simulink library "RxTxFixedPointLibrary_noscopes_org"  (Simulink 10.0)
settings: Solver=VariableStepAuto  StartTime=0.0  StopTime=10.0  RelTol=1e-3
undefined symbols (not defined in the file): AGCBarkerSymbols, coeff, crcDecodeLag, CRCGeneratorLag, EQTrainingSymbols, j, K1, K2, numHeaderBits, numTrainingSamples, pLen, RadioSampleRate, samplesPerSymbol, VibertiTracebackLength, xPreambleSeq
libraries: simulink x33, dsphdlfiltering x20, hdlsllib x13, commseqgen3 x4, dspsigops x4, commdigbbndpm3 x3, commcrc2 x2, commcnvcod2 x2, $bdroot x1, dspstat3 x1, commfilt2 x1
(part 1 of 4)
settings Model: Creator=tcollins  LastModifiedBy=annonymous
settings Model: SuppressorTable=|
  | <?xml version="1.0" encoding="UTF-8" standalone="yes" ?>
  | <!DOCTYPE boost_serialization>
  | <boost_serialization signature="serialization::archive" version="15">
  | <DiagnosticSuppressor class_id="0" tracking_level="0" version="6">
  | 	<Table class_id="1" tracking_level="0" version="0">
  | 		<count>28</count>
  | 		<bucket_count>47</bucket_count>
  | 		<item_version>0</item_version>
  | 		<item class_id="2" tracking_level="0" version="0">
  | 			<first class_id="3" tracking_level="0" version="6">
  | 				<Source class_id="4" tracking_level="0" version="0">
  | 					<count>1</count>
  | 					<item_version>0</item_version>
  | 					<item>RxTxFixedPointLibrary_noscopes_org/Receiver HDL/Frame Recover/Frequency Recovery/Phase Shift FP/Cosine HDL Optimized</item>
  | 				</Source>
  | 			</first>
  | 			<second class_id="5" tracking_level="0" version="6">
  | 				<SuppressedData class_id="6" tracking_level="0" version="0">
  | 					<count>1</count>
  | 					<bucket_count>2</bucket_count>
  | 					<item_version>0</item_version>
  | 					<item class_id="7" tracking_level="0" version="0">
  | 						<first class_id="8" tracking_level="0" version="6">
  | 							<ID>SimulinkFixedPoint:util:fxpParameterPrecisionLoss</ID>
  | 							<Cause>
  | 								<Source>
  | 									<count>0</count>
  | 									<item_version>0</item_version>
  | 								</Source>
  | 							</Cause>
  | 						</first>
  | 						<second class_id="9" tracking_level="0" version="6">
  | 							<Comment></Comment>
  | 							<User></User>
  | 							<LastModified class_id="10" tracking_level="0" version="0">
  | 								<ptime_date class_id="11" tracking_level="0" version="0">
  | 									<date>20160608</date>
  | 								</ptime_date>
  | 								<ptime_time_duration class_id="12" tracking_level="0" version="0">
  | 									<is_special>0</is_special>
  | 									<time_duration_hours>12</time_duration_hours>
  | 									<time_duration_minutes>6</time_duration_minutes>
  | 									<time_duration_seconds>23</time_duration_seconds>
  | 									<time_duration_fractional_seconds>0</time_duration_fractional_seconds>
  | 								</ptime_time_duration>
  | 							</LastModified>
  | 							<SuppressionType>1</SuppressionType>
  | 						</second>
  | 					</item>
  | 				</SuppressedData>
  | 			</second>
  | 		</item>
  | 		<item>
  | 			<first>
  | 				<Source>
  | 					<count>1</count>
  | 					<item_version>0</item_version>
  | 					<item>RxTxFixedPointLibrary_noscopes_org/Receiver HDL/Viterbi Decode/Buffer Frame/FIFO/HDL FIFO4/Upsample2/Counter</item>
  | 				</Source>
  | 			</first>
  | 			<second>
  | 				<SuppressedData>
  | 					<count>2</count>
  | 					<bucket_count>2</bucket_count>
  | 					<item_version>0</item_version>
  | 					<item>
  | 						<first>
  | 							<ID>SimulinkFixedPoint:util:Overflowoccurred</ID>
  | 							<Cause>
  | 								<Source>
  | 									<count>0</count>
  | 									<item_version>0</item_version>
  | 								</Source>
  | 							</Cause>
  | 						</first>
  | 						<second>
  | 							<Comment></Comment>
  | 							<User></User>
  | 							<LastModified>
  | 								<ptime_date>
  | 									<date>20160608</date>
  | 								</ptime_date>
  | 								<ptime_time_duration>
  | 									<is_special>0</is_special>
  | 									<time_duration_hours>15</time_duration_hours>
  | 									<time_duration_minutes>23</time_duration_minutes>
  | 									<time_duration_seconds>17</time_duration_seconds>
  | 									<time_duration_fractional_seconds>0</time_duration_fractional_seconds>
  | 								</ptime_time_duration>
  | 							</LastModified>
  | 							<SuppressionType>1</SuppressionType>
  | 						</second>
  | 					</item>
  | 					<item>
  | 						<first>
  | 							<ID>Simulink:DataType:WarningOverFlowDetected</ID>
  | 							<Cause>
  | 								<Source>
  | 									<count>0</count>
  | 									<item_version>0</item_version>
  | 								</Source>
  | 							</Cause>
  | 						</first>
  | 						<second>
  | 							<Comment></Comment>
  | 							<User></User>
  | 							<LastModified>
  | 								<ptime_date>
  | 									<date>20160608</date>
  | 								</ptime_date>
  | 								<ptime_time_duration>
  | 									<is_special>0</is_special>
  | 									<time_duration_hours>15</time_duration_hours>
  | 									<time_duration_minutes>23</time_duration_minutes>
  | 									<time_duration_seconds>17</time_duration_seconds>
  | 									<time_duration_fractional_seconds>0</time_duration_fractional_seconds>
  | 								</ptime_time_duration>
  | 							</LastModified>
  | 							<SuppressionType>1</SuppressionType>
  | 						</second>
  | 					</item>
  | 				</SuppressedData>
  | 			</second>
  | 		</item>
  | 		<item>
  | 			<first>
  | 				<Source>
  | 					<count>1</count>
  | 					<item_version>0</item_version>
  | 					<item>RxTxFixedPointLibrary_noscopes_org/Transmitter HDL/Packet Generation/Frame Indexer</item>
  | 				</Source>
  | 			</first>
  | 			<second>
  | 				<SuppressedData>
  | 					<count>2</count>
  | 					<bucket_count>2</bucket_count>
  | 					<item_version>0</item_version>
  | 					<item>
  | 						<first>
  | 							<ID>Simulink:DataType:WarningOverFlowDetected</ID>
  | 							<Cause>
  | 								<Source>
  | 									<count>0</count>
  | 									<item_version>0</item_version>
  | 								</Source>
  | 							</Cause>
  | 						</first>
  | 						<second>
  | 							<Comment></Comment>
  | 							<User></User>
  | 							<LastModified>
  | 								<ptime_date>
  | 									<date>20160715</date>
  | 								</ptime_date>
  | 								<ptime_time_duration>
  | 									<is_special>0</is_special>
  | 									<time_duration_hours>14</time_duration_hours>
  | 									<time_duration_minutes>21</time_duration_minutes>
  | 									<time_duration_seconds>36</time_duration_seconds>
  | 									<time_duration_fractional_seconds>0</time_duration_fractional_seconds>
  | 								</ptime_time_duration>
  | 							</LastModified>
  | 							<SuppressionType>1</SuppressionType>
  | 						</second>
  | 					</item>
  | 					<item>
  | 						<first>
  | 							<ID>SimulinkFixedPoint:util:Overflowoccurred</ID>
  | 							<Cause>
  | 								<Source>
  | 									<count>0</count>
  | 									<item_version>0</item_version>
  | 								</Source>
  | 							</Cause>
  | 						</first>
  | 						<second>
  | 							<Comment></Comment>
  | 							<User></User>
  | 							<LastModified>
  | 								<ptime_date>
  | 									<date>20160715</date>
  | 								</ptime_date>
  | 								<ptime_time_duration>
  | 									<is_special>0</is_special>
  | 									<time_duration_hours>14</time_duration_hours>
  | 									<time_duration_minutes>21</time_duration_minutes>
  | 									<time_duration_seconds>36</time_duration_seconds>
  | 									<time_duration_fractional_seconds>0</time_duration_fractional_seconds>
  | 								</ptime_time_duration>
  | 							</LastModified>
  | 							<SuppressionType>1</SuppressionType>
  | 						</second>
  | 					</item>
  | 				</SuppressedData>
  | 			</second>
  | 		</item>
  | 		<item>
  | 			<first>
  | 				<Source>
  | 					<count>1</count>
  | 					<item_version>0</item_version>
  | 					<item>RxTxFixedPointLibrary_noscopes_org/Receiver HDL/Frame Recover/Frequency Recovery/Phase Shift FP/Cosine HDL Optimized/exp hdl/cos_hdl</item>
  | 				</Source>
  | 			</first>
  | 			<second>
  | 				<SuppressedData>
  | 					<count>1</count>
  | 					<bucket_count>2</bucket_count>
  | 					<item_version>0</item_version>
  | 					<item>
  | 						<first>
  | 							<ID>SimulinkFixedPoint:util:fxpParameterPrecisionLoss</ID>
  | 							<Cause>
  | 								<Source>
  | 									<count>0</count>
  | 									<item_version>0</item_version>
  | 								</Source>
  | 							</Cause>
  | 						</first>
  | 						<second>
  | 							<Comment></Comment>
  | 							<User></User>
  | 							<LastModified>
  | 								<ptime_date>
  | 									<date>20160607</date>
  | 								</ptime_date>
  | 								<ptime_time_duration>
  | 									<is_special>0</is_special>
  | 									<time_duration_hours>13</time_duration_hours>
  | 									<time_duration_minutes>40</time_duration_minutes>
  | 									<time_duration_seconds>47</time_duration_seconds>
  | 									<time_duration_fractional_seconds>0</time_duration_fractional_seconds>
  | 								</ptime_time_duration>
  | 							</LastModified>
  | 							<SuppressionType>1</SuppressionType>
  | 						</second>
  | 					</item>
  | 				</SuppressedData>
  | 			</second>
  | 		</item>
  | 		<item>
  | 			<first>
  | 				<Source>
  | 					<count>1</count>
  | 					<item_version>0</item_version>
  | 					<item>RxTxFixedPointLibrary_noscopes_org/Receiver HDL/Frame Recover/Frequency Recovery/Phase Shift FP/Cosine HDL Optimized/exp hdl/sin_hdl/CastU16En3</item>
  | 				</Source>
  | 			</first>
  | 			<second>
  | 				<SuppressedData>
  | 					<count>1</count>
  | 					<bucket_count>2</bucket_count>
  | 					<item_version>0</item_version>
  | 					<item>
  | 						<first>
  | 							<ID>SimulinkFixedPoint:util:Saturationoccurred</ID>
  | 							<Cause>
  | 								<Source>
  | 									<count>0</count>
  | 									<item_version>0</item_version>
  | 								</Source>
  | 							</Cause>
  | 						</first>
  | 						<second>
  | 							<Comment></Comment>
  | 							<User>sdutta</User>
  | 							<LastModified>
  | 								<ptime_date>
  | 									<date>20170912</date>
  | 								</ptime_date>
  | 								<ptime_time_duration>
  | 									<is_special>0</is_special>
  | 									<time_duration_hours>16</time_duration_hours>
  | 									<time_duration_minutes>2</time_duration_minutes>
  | 									<time_duration_seconds>5</time_duration_seconds>
  | 									<time_duration_fractional_seconds>0</time_duration_fractional_seconds>
  | 								</ptime_time_duration>
  | 							</LastModified>
  | 							<SuppressionType>1</SuppressionType>
  | 						</second>
  | 					</item>
  | 				</SuppressedData>
  | 			</second>
  | 		</item>
  | 		<item>
  | 			<first>
  | 				<Source>
  | 					<count>1</count>
  | 					<item_version>0</item_version>
  | 					<item>RxTxFixedPointLibrary_noscopes_org/Transmitter HDL/Packet Generation/Random Data/Unpack/Extract Bits</item>
  | 				</Source>
  | 			</first>
  | 			<second>
  | 				<SuppressedData>
  | 					<count>2</count>
  | 					<bucket_count>2</bucket_count>
  | 					<item_version>0</item_version>
  | 					<item>
  | 						<first>
  | 							<ID>SimulinkFixedPoint:util:Overflowoccurred</ID>
  | 							<Cause>
  | 								<Source>
  | 									<count>0</count>
  | 									<item_version>0</item_version>
  | 								</Source>
  | 							</Cause>
  | 						</first>
  | 						<second>
  | 							<Comment></Comment>
  | 							<User></User>
  | 							<LastModified>
  | 								<ptime_date>
  | 									<date>20160608</date>
  | 								</ptime_date>
  | 								<ptime_time_duration>
  | 									<is_special>0</is_special>
  | 									<time_duration_hours>15</time_duration_hours>
  | 									<time_duration_minutes>43</time_duration_minutes>
  | 									<time_duration_seconds>6</time_duration_seconds>
  | 									<time_duration_fractional_seconds>0</time_duration_fractional_seconds>
  | 								</ptime_time_duration>
  | 							</LastModified>
  | 							<SuppressionType>1</SuppressionType>
  | 						</second>
  | 					</item>
  | 					<item>
  | 						<first>
  | 							<ID>Simulink:DataType:WarningOverFlowDetected</ID>
  | 							<Cause>
  | 								<Source>
  | 									<count>0</count>
  | 									<item_version>0</item_version>
  | 								</Source>
  | 							</Cause>
  | 						</first>
  | 						<second>
  | 							<Comment></Comment>
  | 							<User></User>
  | 							<LastModified>
  | 								<ptime_date>
  | 									<date>20160608</date>
  | 								</ptime_date>
  | 								<ptime_time_duration>
  | 									<is_special>0</is_special>
  | 									<time_duration_hours>15</time_duration_hours>
  | 									<time_duration_minutes>43</time_duration_minutes>
  | 									<time_duration_seconds>6</time_duration_seconds>
  | 									<time_duration_fractional_seconds>0</time_duration_fractional_seconds>
  | 								</ptime_time_duration>
  | 							</LastModified>
  | 							<SuppressionType>1</SuppressionType>
  | 						</second>
  | 					</item>
  | 				</SuppressedData>
  | 			</second>
  | 		</item>
  | 		<item>
  | 			<first>
  | 				<Source>
  | 					<count>1</count>
  | 					<item_version>0</item_version>
  | 					<item>RxTxFixedPointLibrary_noscopes_org/Receiver HDL/Frame Recover/Equalization and Demodulation/DFE/DFE/Map Symbol/HDL Counter</item>
  | 				</Source>
  | 			</first>
  | 			<second>
  | 				<SuppressedData>
  | 					<count>2</count>
  | 					<bucket_count>2</bucket_count>
  | 					<item_version>0</item_version>
  | 					<item>
  | 						<first>
  | 							<ID>Simulink:DataType:WarningOverFlowDetected</ID>
  | 							<Cause>
  | 								<Source>
  | 									<count>0</count>
  | 									<item_version>0</item_version>
  | 								</Source>
  | 							</Cause>
  | 						</first>
  | 						<second>
  | 							<Comment></Comment>
  | 							<User></User>
  | 							<LastModified>
  | 								<ptime_date>
  | 									<date>20160715</date>
  | 								</ptime_date>
  | 								<ptime_time_duration>
  | 									<is_special>0</is_special>
  | 									<time_duration_hours>14</time_duration_hours>
  | 									<time_duration_minutes>21</time_duration_minutes>
  | 									<time_duration_seconds>36</time_duration_seconds>
  | 									<time_duration_fractional_seconds>0</time_duration_fractional_seconds>
  | 								</ptime_time_duration>
  | 							</LastModified>
  | 							<SuppressionType>1</SuppressionType>
  | 						</second>
  | 					</item>
  | 					<item>
  | 						<first>
  | 							<ID>SimulinkFixedPoint:util:Overflowoccurred</ID>
  | 							<Cause>
  | 								<Source>
  | 									<count>0</count>
  | 									<item_version>0</item_version>
  | 								</Source>
  | 							</Cause>
  | 						</first>
  | 						<second>
  | 							<Comment></Comment>
  | 							<User></User>
  | 							<LastModified>
  | 								<ptime_date>
  | 									<date>20160715</date>
  | 								</ptime_date>
  | 								<ptime_time_duration>
  | 									<is_special>0</is_special>
  | 									<time_duration_hours>14</time_duration_hours>
  | 									<time_duration_minutes>21</time_duration_minutes>
  | 									<time_duration_seconds>36</time_duration_seconds>
  | 									<time_duration_fractional_seconds>0</time_duration_fractional_seconds>
  | 								</ptime_time_duration>
  | 							</LastModified>
  | 							<SuppressionType>1</SuppressionType>
  | 						</second>
  | 					</item>
  | 				</SuppressedData>
  | 			</second>
  | 		</item>
  | 		<item>
  | 			<first>
  | 				<Source>
  | 					<count>1</count>
  | 					<item_version>0</item_version>
  | 					<item>RxTxFixedPointLibrary_noscopes_org/Receiver HDL/Viterbi Decode/Buffer Frame/FIFO/HDL FIFO4/Upsample1/Counter</item>
  | 				</Source>
  | 			</first>
  | 			<second>
  | 				<SuppressedData>
  | 					<count>2</count>
  | 					<bucket_count>2</bucket_count>
  | 					<item_version>0</item_version>
  | 					<item>
  | 						<first>
  | 							<ID>SimulinkFixedPoint:util:Overflowoccurred</ID>
  | 							<Cause>
  | 								<Source>
  | 									<count>0</count>
  | 									<item_version>0</item_version>
  | 								</Source>
  | 							</Cause>
  | 						</first>
  | 						<second>
  | 							<Comment></Comment>
  | 							<User></User>
  | 							<LastModified>
  | 								<ptime_date>
  | 									<date>20160608</date>
  | 								</ptime_date>
  | 								<ptime_time_duration>
  | 									<is_special>0</is_special>
  | 									<time_duration_hours>15</time_duration_hours>
  | 									<time_duration_minutes>23</time_duration_minutes>
  | 									<time_duration_seconds>17</time_duration_seconds>
  | 									<time_duration_fractional_seconds>0</time_duration_fractional_seconds>
  | 								</ptime_time_duration>
  | 							</LastModified>
  | 							<SuppressionType>1</SuppressionType>
  | 						</second>
  | 					</item>
  | 					<item>
  | 						<first>
  | 							<ID>Simulink:DataType:WarningOverFlowDetected</ID>
  | 							<Cause>
  | 								<Source>
  | 									<count>0</count>
  | 									<item_version>0</item_version>
  | 								</Source>
  | 							</Cause>
  | 						</first>
  | 						<second>
  | 							<Comment></Comment>
  | 							<User></User>
  | 							<LastModified>
  | 								<ptime_date>
  | 									<date>20160608</date>
  | 								</ptime_date>
  | 								<ptime_time_duration>
  | 									<is_special>0</is_special>
  | 									<time_duration_hours>15</time_duration_hours>
  | 									<time_duration_minutes>23</time_duration_minutes>
  | 									<time_duration_seconds>17</time_duration_seconds>
  | 									<time_duration_fractional_seconds>0</time_duration_fractional_seconds>
  | 								</ptime_time_duration>
  | 							</LastModified>
  | 							<SuppressionType>1</SuppressionType>
  | 						</second>
  | 					</item>
  | 				</SuppressedData>
  | 			</second>
  | 		</item>
  | 		<item>
  | 			<first>
  | 				<Source>
  | 					<count>1</count>
  | 					<item_version>0</item_version>
  | 					<item>RxTxFixedPointLibrary_noscopes_org/Transmitter HDL/Packet Generation/Preamble/HDL Counter</item>
  | 				</Source>
  | 			</first>
  | 			<second>
  | 				<SuppressedData>
  | 					<count>2</count>
  | 					<bucket_count>2</bucket_count>
  | 					<item_version>0</item_version>
  | 					<item>
  | 						<first>
  | 							<ID>Simulink:DataType:WarningOverFlowDetected</ID>
  | 							<Cause>
  | 								<Source>
  | 									<count>0</count>
  | 									<item_version>0</item_version>
  | 								</Source>
  | 							</Cause>
  | 						</first>
  | 						<second>
  | 							<Comment></Comment>
  | 							<User></User>
  | 							<LastModified>
  | 								<ptime_date>
  | 									<date>20160715</date>
  | 								</ptime_date>
  | 								<ptime_time_duration>
  | 									<is_special>0</is_special>
  | 									<time_duration_hours>14</time_duration_hours>
  | 									<time_duration_minutes>21</time_duration_minutes>
  | 									<time_duration_seconds>36</time_duration_seconds>
  | 									<time_duration_fractional_seconds>0</time_duration_fractional_seconds>
  | 								</ptime_time_duration>
  | 							</LastModified>
  | 							<SuppressionType>1</SuppressionType>
  | 						</second>
  | 					</item>
  | 					<item>
  | 						<first>
  | 							<ID>SimulinkFixedPoint:util:Overflowoccurred</ID>
  | 							<Cause>
  | 								<Source>
  | 									<count>0</count>
  | 									<item_version>0</item_version>
  | 								</Source>
  | 							</Cause>
  | 						</first>
  | 						<second>
  | 							<Comment></Comment>
  | 							<User></User>
  | 							<LastModified>
  | 								<ptime_date>
  | 									<date>20160715</date>
  | 								</ptime_date>
  | 								<ptime_time_duration>
  | 									<is_special>0</is_special>
  | 									<time_duration_hours>14</time_duration_hours>
  | 									<time_duration_minutes>21</time_duration_minutes>
  | 									<time_duration_seconds>36</time_duration_seconds>
  | 									<time_duration_fractional_seconds>0</time_duration_fractional_seconds>
  | 								</ptime_time_duration>
  | 							</LastModified>
  | 							<SuppressionType>1</SuppressionType>
  | 						</second>
  | 					</item>
  | 				</SuppressedData>
  | 			</second>
  | 		</item>
  | 		<item>
  | 			<first>
  | 				<Source>
  | 					<count>1</count>
  | 					<item_version>0</item_version>
  | 					<item>RxTxFixedPointLibrary_noscopes_org/Transmitter HDL/Packet Generation/Random Data/Unpack/Extract Bits1</item>
  | 				</Source>
  | 			</first>
  | 			<second>
  | 				<SuppressedData>
  | 					<count>2</count>
  | 					<bucket_count>2</bucket_count>
  | 					<item_version>0</item_version>
  | 					<item>
  | 						<first>
  | 							<ID>SimulinkFixedPoint:util:Overflowoccurred</ID>
  | 							<Cause>
  | 								<Source>
  | 									<count>0</count>
  | 									<item_version>0</item_version>
  | 								</Source>
  | 							</Cause>
  | 						</first>
  | 						<second>
  | 							<Comment></Comment>
  | 							<User></User>
  | 							<LastModified>
  | 								<ptime_date>
  | 									<date>20160608</date>
  | 								</ptime_date>
  | 								<ptime_time_duration>
  | 									<is_special>0</is_special>
  | 									<time_duration_hours>15</time_duration_hours>
  | 									<time_duration_minutes>43</time_duration_minutes>
  | 									<time_duration_seconds>6</time_duration_seconds>
  | 									<time_duration_fractional_seconds>0</time_duration_fractional_seconds>
  | 								</ptime_time_duration>
  | 							</LastModified>
  | 							<SuppressionType>1</SuppressionType>
  | 						</second>
  | 					</item>
  | 					<item>
  | 						<first>
  | 							<ID>Simulink:DataType:WarningOverFlowDetected</ID>
  | 							<Cause>
  | 								<Source>
  | 									<count>0</count>
  | 									<item_version>0</item_version>
  | 								</Source>
  | 							</Cause>
  | 						</first>
  | 						<second>
  | 							<Comment></Comment>
  | 							<User></User>
  | 							<LastModified>
  | 								<ptime_date>
  | 									<date>20160608</date>
  | 								</ptime_date>
  | 								<ptime_time_duration>
  | 									<is_special>0</is_special>
  | 									<time_duration_hours>15</time_duration_hours>
  | 									<time_duration_minutes>43</time_duration_minutes>
  | 									<time_duration_seconds>6</time_duration_seconds>
  | 									<time_duration_fractional_seconds>0</time_duration_fractional_seconds>
  | 								</ptime_time_duration>
  | 							</LastModified>
  | 							<SuppressionType>1</SuppressionType>
  | 						</second>
  | 					</item>
  | 				</SuppressedData>
  | 			</second>
  | 		</item>
  | 		<item>
  | 			<first>
  | 				<Source>
  | 					<count>1</count>
  | 					<item_version>0</item_version>
  | 					<item>RxTxFixedPointLibrary_noscopes_org/Receiver HDL/Frame Recover/Frequency Recovery/Phase Shift FP/Cosine HDL Optimized/exp hdl/sin_hdl/insig</item>
  | 				</Source>
  | 			</first>
  | 			<second>
  | 				<SuppressedData>
  | 					<count>1</count>
  | 					<bucket_count>2</bucket_count>
  | 					<item_version>0</item_version>
  | 					<item>
  | 						<first>
  | 							<ID>SimulinkFixedPoint:util:Overflowoccurred</ID>
  | 							<Cause>
  | 								<Source>
  | 									<count>0</count>
  | 									<item_version>0</item_version>
  | 								</Source>
  | 							</Cause>
  | 						</first>
  | 						<second>
  | 							<Comment></Comment>
  | 							<User>sdutta</User>
  | 							<LastModified>
  | 								<ptime_date>
  | 									<date>20170912</date>
  | 								</ptime_date>
  | 								<ptime_time_duration>
  | 									<is_special>0</is_special>
  | 									<time_duration_hours>16</time_duration_hours>
  | 									<time_duration_minutes>2</time_duration_minutes>
  | 									<time_duration_seconds>5</time_duration_seconds>
  | 									<time_duration_fractional_seconds>0</time_duration_fractional_seconds>
  | 								</ptime_time_duration>
  | 							</LastModified>
  | 							<SuppressionType>1</SuppressionType>
  | 						</second>
  | 					</item>
  | 				</SuppressedData>
  | 			</second>
  | 		</item>
  | 		<item>
  | 			<first>
  | 				<Source>
  | 					<count>1</count>
  | 					<item_version>0</item_version>
  | 					<item>RxTxFixedPointLibrary_noscopes_org/Receiver HDL/Viterbi Decode/Buffer Frame/FIFO/HDL FIFO3/Upsample/Counter</item>
  | 				</Source>
  | 			</first>
  | 			<second>
  | 				<SuppressedData>
  | 					<count>2</count>
  | 					<bucket_count>2</bucket_count>
  | 					<item_version>0</item_version>
  | 					<item>
  | 						<first>
  | 							<ID>Simulink:DataType:WarningOverFlowDetected</ID>
  | 							<Cause>
  | 								<Source>
  | 									<count>0</count>
  | 									<item_version>0</item_version>
  | 								</Source>
  | 							</Cause>
  | 						</first>
  | 						<second>
  | 							<Comment></Comment>
  | 							<User></User>
  | 							<LastModified>
  | 								<ptime_date>
  | 									<date>20160608</date>
  | 								</ptime_date>
  | 								<ptime_time_duration>
  | 									<is_special>0</is_special>
  | 									<time_duration_hours>15</time_duration_hours>
  | 									<time_duration_minutes>23</time_duration_minutes>
  | 									<time_duration_seconds>17</time_duration_seconds>
  | 									<time_duration_fractional_seconds>0</time_duration_fractional_seconds>
  | 								</ptime_time_duration>
  | 							</LastModified>
  | 							<SuppressionType>1</SuppressionType>
  | 						</second>
  | 					</item>
  | 					<item>
  | 						<first>
  | 							<ID>SimulinkFixedPoint:util:Overflowoccurred</ID>
  | 							<Cause>
  | 								<Source>
  | 									<count>0</count>
  | 									<item_version>0</item_version>
  | 								</Source>
  | 							</Cause>
  | 						</first>
  | 						<second>
  | 							<Comment></Comment>
  | 							<User></User>
  | 							<LastModified>
  | 								<ptime_date>
  | 									<date>20160608</date>
  | 								</ptime_date>
  | 								<ptime_time_duration>
  | 									<is_special>0</is_special>
  | 									<time_duration_hours>15</time_duration_hours>
  | 									<time_duration_minutes>23</time_duration_minutes>
  | 									<time_duration_seconds>17</time_duration_seconds>
  | 									<time_duration_fractional_seconds>0</time_duration_fractional_seconds>
  | 								</ptime_time_duration>
  | 							</LastModified>
  | 							<SuppressionType>1</SuppressionType>
  | 						</second>
  | 					</item>
  | 				</SuppressedData>
  | 			</second>
  | 		</item>
  | 		<item>
  | 			<first>
  | 				<Source>
  | 					<count>1</count>
  | 					<item_version>0</item_version>
  | 					<item>RxTxFixedPointLibrary_noscopes_org/Transmitter HDL/Packet Generation/Preamble/Unpack1/Extract Bits</item>
  | 				</Source>
  | 			</first>
  | 			<second>
  | 				<SuppressedData>
  | 					<count>2</count>
  | 					<bucket_count>2</bucket_count>
  | 					<item_version>0</item_version>
  | 					<item>
  | 						<first>
  | 							<ID>SimulinkFixedPoint:util:Overflowoccurred</ID>
  | 							<Cause>
  | 								<Source>
  | 									<count>0</count>
  | 									<item_version>0</item_version>
  | 								</Source>
  | 							</Cause>
  | 						</first>
  | 						<second>
  | 							<Comment></Comment>
  | 							<User></User>
  | 							<LastModified>
  | 								<ptime_date>
  | 									<date>20160608</date>
  | 								</ptime_date>
  | 								<ptime_time_duration>
  | 									<is_special>0</is_special>
  | 									<time_duration_hours>15</time_duration_hours>
  | 									<time_duration_minutes>43</time_duration_minutes>
  | 									<time_duration_seconds>6</time_duration_seconds>
  | 									<time_duration_fractional_seconds>0</time_duration_fractional_seconds>
  | 								</ptime_time_duration>
  | 							</LastModified>
  | 							<SuppressionType>1</SuppressionType>
  | 						</second>
  | 					</item>
  | 					<item>
  | 						<first>
  | 							<ID>Simulink:DataType:WarningOverFlowDetected</ID>
  | 							<Cause>
  | 								<Source>
  | 									<count>0</count>
  | 									<item_version>0</item_version>
  | 								</Source>
  | 							</Cause>
  | 						</first>
  | 						<second>
  | 							<Comment></Comment>
  | 							<User></User>
  | 							<LastModified>
  | 								<ptime_date>
  | 									<date>20160608</date>
  | 								</ptime_date>
  | 								<ptime_time_duration>
  | 									<is_special>0</is_special>
  | 									<time_duration_hours>15</time_duration_hours>
  | 									<time_duration_minutes>43</time_duration_minutes>
  | 									<time_duration_seconds>6</time_duration_seconds>
  | 									<time_duration_fractional_seconds>0</time_duration_fractional_seconds>
  | 								</ptime_time_duration>
  | 							</LastModified>
  | 							<SuppressionType>1</SuppressionType>
  | 						</second>
  | 					</item>
  | 				</SuppressedData>
  | 			</second>
  | 		</item>
  | 		<item>
  | 			<first>
  | 				<Source>
  | 					<count>1</count>
  | 					<item_version>0</item_version>
  | 					<item>RxTxFixedPointLibrary_noscopes_org/Receiver HDL/Frame Recover/Manage Error Signals/Peak Detector Counter</item>
  | 				</Source>
  | 			</first>
  | 			<second>
  | 				<SuppressedData>
  | 					<count>2</count>
  | 					<bucket_count>2</bucket_count>
  | 					<item_version>0</item_version>
  | 					<item>
  | 						<first>
  | 							<ID>SimulinkFixedPoint:util:Overflowoccurred</ID>
  | 							<Cause>
  | 								<Source>
  | 									<count>0</count>
  | 									<item_version>0</item_version>
  | 								</Source>
  | 							</Cause>
  | 						</first>
  | 						<second>
  | 							<Comment></Comment>
  | 							<User></User>
  | 							<LastModified>
  | 								<ptime_date>
  | 									<date>20160715</date>
  | 								</ptime_date>
  | 								<ptime_time_duration>
  | 									<is_special>0</is_special>
  | 									<time_duration_hours>14</time_duration_hours>
  | 									<time_duration_minutes>21</time_duration_minutes>
  | 									<time_duration_seconds>36</time_duration_seconds>
  | 									<time_duration_fractional_seconds>0</time_duration_fractional_seconds>
  | 								</ptime_time_duration>
  | 							</LastModified>
  | 							<SuppressionType>1</SuppressionType>
  | 						</second>
  | 					</item>
  | 					<item>
  | 						<first>
  | 							<ID>Simulink:DataType:WarningOverFlowDetected</ID>
  | 							<Cause>
  | 								<Source>
  | 									<count>0</count>
  | 									<item_version>0</item_version>
  | 								</Source>
  | 							</Cause>
  | 						</first>
  | 						<second>
  | 							<Comment></Comment>
  | 							<User></User>
  | 							<LastModified>
  | 								<ptime_date>
  | 									<date>20160715</date>
  | 								</ptime_date>
  | 								<ptime_time_duration>
  | 									<is_special>0</is_special>
  | 									<time_duration_hours>14</time_duration_hours>
  | 									<time_duration_minutes>21</time_duration_minutes>
  | 									<time_duration_seconds>36</time_duration_seconds>
  | 									<time_duration_fractional_seconds>0</time_duration_fractional_seconds>
  | 								</ptime_time_duration>
  | 							</LastModified>
  | 							<SuppressionType>1</SuppressionType>
  | 						</second>
  | 					</item>
  | 				</SuppressedData>
  | 			</second>
  | 		</item>
  | 		<item>
  | 			<first>
  | 				<Source>
  | 					<count>1</count>
  | 					<item_version>0</item_version>
  | 					<item>RxTxFixedPointLibrary_noscopes_org/Receiver HDL/Frame Recover/Frequency Recovery/Phase Shift FP/Cosine HDL Optimized/exp hdl/cos_hdl/insig</item>
  | 				</Source>
  | 			</first>
  | 			<second>
  | 				<SuppressedData>
  | 					<count>1</count>
  | 					<bucket_count>2</bucket_count>
  | 					<item_version>0</item_version>
  | 					<item>
  | 						<first>
  | 							<ID>SimulinkFixedPoint:util:Overflowoccurred</ID>
  | 							<Cause>
  | 								<Source>
  | 									<count>0</count>
  | 									<item_version>0</item_version>
  | 								</Source>
  | 							</Cause>
  | 						</first>
  | 						<second>
  | 							<Comment></Comment>
  | 							<User>sdutta</User>
  | 							<LastModified>
  | 								<ptime_date>
  | 									<date>20170912</date>
  | 								</ptime_date>
  | 								<ptime_time_duration>
  | 									<is_special>0</is_special>
  | 									<time_duration_hours>16</time_duration_hours>
  | 									<time_duration_minutes>2</time_duration_minutes>
  | 									<time_duration_seconds>5</time_duration_seconds>
  | 									<time_duration_fractional_seconds>0</time_duration_fractional_seconds>
  | 								</ptime_time_duration>
  | 							</LastModified>
  | 							<SuppressionType>1</SuppressionType>
  | 						</second>
  | 					</item>
  | 				</SuppressedData>
  | 			</second>
  | 		</item>
  | 		<item>
  | 			<first>
  | 				<Source>
  | 					<count>1</count>
  | 					<item_version>0</item_version>
  | 					<item>RxTxFixedPointLibrary_noscopes_org/Receiver HDL/CRC Check and DMA Pack/Debug Selector/Packet Counter</item>
  | 				</Source>
  | 			</first>
  | 			<second>
  | 				<SuppressedData>
  | 					<count>2</count>
  | 					<bucket_count>2</bucket_count>
  | 					<item_version>0</item_version>
  | 					<item>
  | 						<first>
  | 							<ID>SimulinkFixedPoint:util:Overflowoccurred</ID>
  | 							<Cause>
  | 								<Source>
  | 									<count>0</count>
  | 									<item_version>0</item_version>
  | 								</Source>
  | 							</Cause>
  | 						</first>
  | 						<second>
  | 							<Comment></Comment>
  | 							<User></User>
  | 							<LastModified>
  | 								<ptime_date>
  | 									<date>20160715</date>
  | 								</ptime_date>
  | 								<ptime_time_duration>
  | 									<is_special>0</is_special>
  | 									<time_duration_hours>14</time_duration_hours>
  | 									<time_duration_minutes>21</time_duration_minutes>
  | 									<time_duration_seconds>36</time_duration_seconds>
  | 									<time_duration_fractional_seconds>0</time_duration_fractional_seconds>
  | 								</ptime_time_duration>
  | 							</LastModified>
  | 							<SuppressionType>1</SuppressionType>
  | 						</second>
  | 					</item>
  | 					<item>
  | 						<first>
  | 							<ID>Simulink:DataType:WarningOverFlowDetected</ID>
  | 							<Cause>
  | 								<Source>
  | 									<count>0</count>
  | 									<item_version>0</item_version>
  | 								</Source>
  | 							</Cause>
  | 						</first>
  | 						<second>
  | 							<Comment></Comment>
  | 							<User></User>
  | 							<LastModified>
  | 								<ptime_date>
  | 									<date>20160715</date>
  | 								</ptime_date>
  | 								<ptime_time_duration>
  | 									<is_special>0</is_special>
  | 									<time_duration_hours>14</time_duration_hours>
  | 									<time_duration_minutes>21</time_duration_minutes>
  | 									<time_duration_seconds>36</time_duration_seconds>
  | 									<time_duration_fractional_seconds>0</time_duration_fractional_seconds>
  | 								</ptime_time_duration>
  | 							</LastModified>
  | 							<SuppressionType>1</SuppressionType>
  | 						</second>
  | 					</item>
  | 				</SuppressedData>
  | 			</second>
  | 		</item>
  | 		<item>
  | 			<first>
  | 				<Source>
  | 					<count>1</count>
  | 					<item_version>0</item_version>
  | 					<item>RxTxFixedPointLibrary_noscopes_org/Receiver HDL/Viterbi Decode/Buffer Frame/HDL Counter</item>
  | 				</Source>
  | 			</first>
  | 			<second>
  | 				<SuppressedData>
  | 					<count>2</count>
  | 					<bucket_count>2</bucket_count>
  | 					<item_version>0</item_version>
  | 					<item>
  | 						<first>
  | 							<ID>Simulink:DataType:WarningOverFlowDetected</ID>
  | 							<Cause>
  | 								<Source>
  | 									<count>0</count>
  | 									<item_version>0</item_version>
  | 								</Source>
  | 							</Cause>
  | 						</first>
  | 						<second>
  | 							<Comment></Comment>
  | 							<User></User>
  | 							<LastModified>
  | 								<ptime_date>
  | 									<date>20160715</date>
  | 								</ptime_date>
  | 								<ptime_time_duration>
  | 									<is_special>0</is_special>
  | 									<time_duration_hours>14</time_duration_hours>
  | 									<time_duration_minutes>21</time_duration_minutes>
  | 									<time_duration_seconds>36</time_duration_seconds>
  | 									<time_duration_fractional_seconds>0</time_duration_fractional_seconds>
  | 								</ptime_time_duration>
  | 							</LastModified>
  | 							<SuppressionType>1</SuppressionType>
  | 						</second>
  | 					</item>
  | 					<item>
  | 						<first>
  | 							<ID>SimulinkFixedPoint:util:Overflowoccurred</ID>
  | 							<Cause>
  | 								<Source>
  | 									<count>0</count>
  | 									<item_version>0</item_version>
  | 								</Source>
  | 							</Cause>
  | 						</first>
  | 						<second>
  | 							<Comment></Comment>
  | 							<User></User>
  | 							<LastModified>
  | 								<ptime_date>
  | 									<date>20160715</date>
  | 								</ptime_date>
  | 								<ptime_time_duration>
  | 									<is_special>0</is_special>
  | 									<time_duration_hours>14</time_duration_hours>
  | 									<time_duration_minutes>21</time_duration_minutes>
  | 									<time_duration_seconds>36</time_duration_seconds>
  | 									<time_duration_fractional_seconds>0</time_duration_fractional_seconds>
  | 								</ptime_time_duration>
  | 							</LastModified>
  | 							<SuppressionType>1</SuppressionType>
  | 						</second>
  | 					</item>
  | 				</SuppressedData>
  | 			</second>
  | 		</item>
  | 		<item>
  | 			<first>
  | 				<Source>
  | 					<count>1</count>
  | 					<item_version>0</item_version>
  | 					<item>RxTxFixedPointLibrary_noscopes_org/Transmitter HDL/Packet Generation/Preamble/Unpack1/Extract Bits1</item>
  | 				</Source>
  | 			</first>
  | 			<second>
  | 				<SuppressedData>
  | 					<count>2</count>
  | 					<bucket_count>2</bucket_count>
  | 					<item_version>0</item_version>
  | 					<item>
  | 						<first>
  | 							<ID>SimulinkFixedPoint:util:Overflowoccurred</ID>
  | 							<Cause>
  | 								<Source>
  | 									<count>0</count>
  | 									<item_version>0</item_version>
  | 								</Source>
  | 							</Cause>
  | 						</first>
  | 						<second>
  | 							<Comment></Comment>
  | 							<User></User>
  | 							<LastModified>
  | 								<ptime_date>
  | 									<date>20160608</date>
  | 								</ptime_date>
  | 								<ptime_time_duration>
  | 									<is_special>0</is_special>
  | 									<time_duration_hours>15</time_duration_hours>
  | 									<time_duration_minutes>43</time_duration_minutes>
  | 									<time_duration_seconds>6</time_duration_seconds>
  | 									<time_duration_fractional_seconds>0</time_duration_fractional_seconds>
  | 								</ptime_time_duration>
  | 							</LastModified>
  | 							<SuppressionType>1</SuppressionType>
  | 						</second>
  | 					</item>
  | 					<item>
  | 						<first>
  | 							<ID>Simulink:DataType:WarningOverFlowDetected</ID>
  | 							<Cause>
  | 								<Source>
  | 									<count>0</count>
  | 									<item_version>0</item_version>
  | 								</Source>
  | 							</Cause>
  | 						</first>
  | 						<second>
  | 							<Comment></Comment>
  | 							<User></User>
  | 							<LastModified>
  | 								<ptime_date>
  | 									<date>20160608</date>
  | 								</ptime_date>
  | 								<ptime_time_duration>
  | 									<is_special>0</is_special>
  | 									<time_duration_hours>15</time_duration_hours>
  | 									<time_duration_minutes>43</time_duration_minutes>
  | 									<time_duration_seconds>6</time_duration_seconds>
  | 									<time_duration_fractional_seconds>0</time_duration_fractional_seconds>
  | 								</ptime_time_duration>
  | 							</LastModified>
  | 							<SuppressionType>1</SuppressionType>
  | 						</second>
  | 					</item>
  | 				</SuppressedData>
  | 			</second>
  | 		</item>
  | 		<item>
  | 			<first>
  | 				<Source>
  | 					<count>1</count>
  | 					<item_version>0</item_version>
  | 					<item>RxTxFixedPointLibrary_noscopes_org/Receiver HDL/Viterbi Decode/Buffer Frame/Check Packet Size/HDL Counter1</item>
  | 				</Source>
  | 			</first>
  | 			<second>
  | 				<SuppressedData>
  | 					<count>2</count>
  | 					<bucket_count>2</bucket_count>
  | 					<item_version>0</item_version>
  | 					<item>
  | 						<first>
  | 							<ID>SimulinkFixedPoint:util:Overflowoccurred</ID>
  | 							<Cause>
  | 								<Source>
  | 									<count>0</count>
  | 									<item_version>0</item_version>
  | 								</Source>
  | 							</Cause>
  | 						</first>
  | 						<second>
  | 							<Comment></Comment>
  | 							<User></User>
  | 							<LastModified>
  | 								<ptime_date>
  | 									<date>20160715</date>
  | 								</ptime_date>
  | 								<ptime_time_duration>
  | 									<is_special>0</is_special>
  | 									<time_duration_hours>14</time_duration_hours>
  | 									<time_duration_minutes>21</time_duration_minutes>
  | 									<time_duration_seconds>36</time_duration_seconds>
  | 									<time_duration_fractional_seconds>0</time_duration_fractional_seconds>
  | 								</ptime_time_duration>
  | 							</LastModified>
  | 							<SuppressionType>1</SuppressionType>
  | 						</second>
  | 					</item>
  | 					<item>
  | 						<first>
  | 							<ID>Simulink:DataType:WarningOverFlowDetected</ID>
  | 							<Cause>
  | 								<Source>
  | 									<count>0</count>
  | 									<item_version>0</item_version>
  | 								</Source>
  | 							</Cause>
  | 						</first>
  | 						<second>
  | 							<Comment></Comment>
  | 							<User></User>
  | 							<LastModified>
  | 								<ptime_date>
  | 									<date>20160715</date>
  | 								</ptime_date>
  | 								<ptime_time_duration>
  | 									<is_special>0</is_special>
  | 									<time_duration_hours>14</time_duration_hours>
  | 									<time_duration_minutes>21</time_duration_minutes>
  | 									<time_duration_seconds>36</time_duration_seconds>
  | 									<time_duration_fractional_seconds>0</time_duration_fractional_seconds>
  | 								</ptime_time_duration>
  | 							</LastModified>
  | 							<SuppressionType>1</SuppressionType>
  | 						</second>
  | 					</item>
  | 				</SuppressedData>
  | 			</second>
  | 		</item>
  | 		<item>
  | 			<first>
  | 				<Source>
  | 					<count>1</count>
  | 					<item_version>0</item_version>
  | 					<item>RxTxFixedPointLibrary_noscopes_org/Receiver HDL/Viterbi Decode/Buffer Frame/FIFO/HDL FIFO4/Upsample/Counter</item>
  | 				</Source>
  | 			</first>
  | 			<second>
  | 				<SuppressedData>
  | 					<count>2</count>
  | 					<bucket_count>2</bucket_count>
  | 					<item_version>0</item_version>
  | 					<item>
  | 						<first>
  | 							<ID>SimulinkFixedPoint:util:Overflowoccurred</ID>
  | 							<Cause>
  | 								<Source>
  | 									<count>0</count>
  | 									<item_version>0</item_version>
  | 								</Source>
  | 							</Cause>
  | 						</first>
  | 						<second>
  | 							<Comment></Comment>
  | 							<User></User>
  | 							<LastModified>
  | 								<ptime_date>
  | 									<date>20160608</date>
  | 								</ptime_date>
  | 								<ptime_time_duration>
  | 									<is_special>0</is_special>
  | 									<time_duration_hours>15</time_duration_hours>
  | 									<time_duration_minutes>23</time_duration_minutes>
  | 									<time_duration_seconds>17</time_duration_seconds>
  | 									<time_duration_fractional_seconds>0</time_duration_fractional_seconds>
  | 								</ptime_time_duration>
  | 							</LastModified>
  | 							<SuppressionType>1</SuppressionType>
  | 						</second>
  | 					</item>
  | 					<item>
  | 						<first>
  | 							<ID>Simulink:DataType:WarningOverFlowDetected</ID>
  | 							<Cause>
  | 								<Source>
  | 									<count>0</count>
  | 									<item_version>0</item_version>
  | 								</Source>
  | 							</Cause>
  | 						</first>
  | 						<second>
  | 							<Comment></Comment>
  | 							<User></User>
  | 							<LastModified>
  | 								<ptime_date>
  | 									<date>20160608</date>
  | 								</ptime_date>
  | 								<ptime_time_duration>
  | 									<is_special>0</is_special>
  | 									<time_duration_hours>15</time_duration_hours>
  | 									<time_duration_minutes>23</time_duration_minutes>
  | 									<time_duration_seconds>17</time_duration_seconds>
  | 									<time_duration_fractional_seconds>0</time_duration_fractional_seconds>
  | 								</ptime_time_duration>
  | 							</LastModified>
  | 							<SuppressionType>1</SuppressionType>
  | 						</second>
  | 					</item>
  | 				</SuppressedData>
  | 			</second>
  | 		</item>
  | 		<item>
  | 			<first>
  | 				<Source>
  | 					<count>1</count>
  | 					<item_version>0</item_version>
  | 					<item>RxTxFixedPointLibrary_noscopes_org/Receiver HDL/Frame Recover/Frequency Recovery/Phase Shift FP/Cosine HDL Optimized/exp hdl/cos_hdl/CastU16En2</item>
  | 				</Source>
  | 			</first>
  | 			<second>
  | 				<SuppressedData>
  | 					<count>1</count>
  | 					<bucket_count>2</bucket_count>
  | 					<item_version>0</item_version>
  | 					<item>
  | 						<first>
  | 							<ID>SimulinkFixedPoint:util:Saturationoccurred</ID>
  | 							<Cause>
  | 								<Source>
  | 									<count>0</count>
  | 									<item_version>0</item_version>
  | 								</Source>
  | 							</Cause>
  | 						</first>
  | 						<second>
  | 							<Comment></Comment>
  | 							<User>sdutta</User>
  | 							<LastModified>
  | 								<ptime_date>
  | 									<date>20170912</date>
  | 								</ptime_date>
  | 								<ptime_time_duration>
  | 									<is_special>0</is_special>
  | 									<time_duration_hours>16</time_duration_hours>
  | 									<time_duration_minutes>2</time_duration_minutes>
  | 									<time_duration_seconds>5</time_duration_seconds>
  | 									<time_duration_fractional_seconds>0</time_duration_fractional_seconds>
  | 								</ptime_time_duration>
  | 							</LastModified>
  | 							<SuppressionType>1</SuppressionType>
  | 						</second>
  | 					</item>
  | 				</SuppressedData>
  | 			</second>
  | 		</item>
  | 		<item>
  | 			<first>
  | 				<Source>
  | 					<count>1</count>
  | 					<item_version>0</item_version>
  | 					<item>RxTxFixedPointLibrary_noscopes_org/Receiver HDL/CRC Check and DMA Pack/Debug Selector/CRC Counter</item>
  | 				</Source>
  | 			</first>
  | 			<second>
  | 				<SuppressedData>
  | 					<count>2</count>
  | 					<bucket_count>2</bucket_count>
  | 					<item_version>0</item_version>
  | 					<item>
  | 						<first>
  | 							<ID>SimulinkFixedPoint:util:Overflowoccurred</ID>
  | 							<Cause>
  | 								<Source>
  | 									<count>0</count>
  | 									<item_version>0</item_version>
  | 								</Source>
  | 							</Cause>
  | 						</first>
  | 						<second>
  | 							<Comment></Comment>
  | 							<User></User>
  | 							<LastModified>
  | 								<ptime_date>
  | 									<date>20160715</date>
  | 								</ptime_date>
  | 								<ptime_time_duration>
  | 									<is_special>0</is_special>
  | 									<time_duration_hours>14</time_duration_hours>
  | 									<time_duration_minutes>21</time_duration_minutes>
  | 									<time_duration_seconds>36</time_duration_seconds>
  | 									<time_duration_fractional_seconds>0</time_duration_fractional_seconds>
  | 								</ptime_time_duration>
  | 							</LastModified>
  | 							<SuppressionType>1</SuppressionType>
  | 						</second>
  | 					</item>
  | 					<item>
  | 						<first>
  | 							<ID>Simulink:DataType:WarningOverFlowDetected</ID>
  | 							<Cause>
  | 								<Source>
  | 									<count>0</count>
  | 									<item_version>0</item_version>
  | 								</Source>
  | 							</Cause>
  | 						</first>
  | 						<second>
  | 							<Comment></Comment>
  | 							<User></User>
  | 							<LastModified>
  | 								<ptime_date>
  | 									<date>20160715</date>
  | 								</ptime_date>
  | 								<ptime_time_duration>
  | 									<is_special>0</is_special>
  | 									<time_duration_hours>14</time_duration_hours>
  | 									<time_duration_minutes>21</time_duration_minutes>
  | 									<time_duration_seconds>36</time_duration_seconds>
  | 									<time_duration_fractional_seconds>0</time_duration_fractional_seconds>
  | 								</ptime_time_duration>
  | 							</LastModified>
  | 							<SuppressionType>1</SuppressionType>
  | 						</second>
  | 					</item>
  | 				</SuppressedData>
  | 			</second>
  | 		</item>
  | 		<item>
  | 			<first>
  | 				<Source>
  | 					<count>1</count>
  | 					<item_version>0</item_version>
  | 					<item>RxTxFixedPointLibrary_noscopes_org/Receiver HDL/Viterbi Decode/Buffer Frame/FIFO/HDL FIFO3/Upsample1/Counter</item>
  | 				</Source>
  | 			</first>
  | 			<second>
  | 				<SuppressedData>
  | 					<count>2</count>
  | 					<bucket_count>2</bucket_count>
  | 					<item_version>0</item_version>
  | 					<item>
  | 						<first>
  | 							<ID>Simulink:DataType:WarningOverFlowDetected</ID>
  | 							<Cause>
  | 								<Source>
  | 									<count>0</count>
  | 									<item_version>0</item_version>
  | 								</Source>
  | 							</Cause>
  | 						</first>
  | 						<second>
  | 							<Comment></Comment>
  | 							<User></User>
  | 							<LastModified>
  | 								<ptime_date>
  | 									<date>20160608</date>
  | 								</ptime_date>
  | 								<ptime_time_duration>
  | 									<is_special>0</is_special>
  | 									<time_duration_hours>15</time_duration_hours>
  | 									<time_duration_minutes>23</time_duration_minutes>
  | 									<time_duration_seconds>17</time_duration_seconds>
  | 									<time_duration_fractional_seconds>0</time_duration_fractional_seconds>
  | 								</ptime_time_duration>
  | 							</LastModified>
  | 							<SuppressionType>1</SuppressionType>
  | 						</second>
  | 					</item>
  | 					<item>
  | 						<first>
  | 							<ID>SimulinkFixedPoint:util:Overflowoccurred</ID>
  | 							<Cause>
  | 								<Source>
  | 									<count>0</count>
  | 									<item_version>0</item_version>
  | 								</Source>
  | 							</Cause>
  | 						</first>
  | 						<second>
  | 							<Comment></Comment>
  | 							<User></User>
  | 							<LastModified>
  | 								<ptime_date>
  | 									<date>20160608</date>
  | 								</ptime_date>
  | 								<ptime_time_duration>
  | 									<is_special>0</is_special>
  | 									<time_duration_hours>15</time_duration_hours>
  | 									<time_duration_minutes>23</time_duration_minutes>
  | 									<time_duration_seconds>17</time_duration_seconds>
  | 									<time_duration_fractional_seconds>0</time_duration_fractional_seconds>
  | 								</ptime_time_duration>
  | 							</LastModified>
  | 							<SuppressionType>1</SuppressionType>
  | 						</second>
  | 					</item>
  | 				</SuppressedData>
  | 			</second>
  | 		</item>
  | 		<item>
  | 			<first>
  | 				<Source>
  | 					<count>1</count>
  | 					<item_version>0</item_version>
  | 					<item>RxTxFixedPointLibrary_noscopes_org/Receiver HDL/Frame Recover/Manage Error Signals/Header Failure Counter</item>
  | 				</Source>
  | 			</first>
  | 			<second>
  | 				<SuppressedData>
  | 					<count>2</count>
  | 					<bucket_count>2</bucket_count>
  | 					<item_version>0</item_version>
  | 					<item>
  | 						<first>
  | 							<ID>Simulink:DataType:WarningOverFlowDetected</ID>
  | 							<Cause>
  | 								<Source>
  | 									<count>0</count>
  | 									<item_version>0</item_version>
  | 								</Source>
  | 							</Cause>
  | 						</first>
  | 						<second>
  | 							<Comment></Comment>
  | 							<User></User>
  | 							<LastModified>
  | 								<ptime_date>
  | 									<date>20160715</date>
  | 								</ptime_date>
  | 								<ptime_time_duration>
  | 									<is_special>0</is_special>
  | 									<time_duration_hours>14</time_duration_hours>
  | 									<time_duration_minutes>21</time_duration_minutes>
  | 									<time_duration_seconds>36</time_duration_seconds>
  | 									<time_duration_fractional_seconds>0</time_duration_fractional_seconds>
  | 								</ptime_time_duration>
  | 							</LastModified>
  | 							<SuppressionType>1</SuppressionType>
  | 						</second>
  | 					</item>
  | 					<item>
  | 						<first>
  | 							<ID>SimulinkFixedPoint:util:Overflowoccurred</ID>
  | 							<Cause>
  | 								<Source>
  | 									<count>0</count>
  | 									<item_version>0</item_version>
  | 								</Source>
  | 							</Cause>
  | 						</first>
  | 						<second>
  | 							<Comment></Comment>
  | 							<User></User>
  | 							<LastModified>
  | 								<ptime_date>
  | 									<date>20160715</date>
  | 								</ptime_date>
  | 								<ptime_time_duration>
  | 									<is_special>0</is_special>
  | 									<time_duration_hours>14</time_duration_hours>
  | 									<time_duration_minutes>21</time_duration_minutes>
  | 									<time_duration_seconds>36</time_duration_seconds>
  | 									<time_duration_fractional_seconds>0</time_duration_fractional_seconds>
  | 								</ptime_time_duration>
  | 							</LastModified>
  | 							<SuppressionType>1</SuppressionType>
  | 						</second>
  | 					</item>
  | 				</SuppressedData>
  | 			</second>
  | 		</item>
  | 		<item>
  | 			<first>
  | 				<Source>
  | 					<count>1</count>
  | 					<item_version>0</item_version>
  | 					<item>RxTxFixedPointLibrary_noscopes_org/Receiver HDL/Viterbi Decode/Buffer Frame/FIFO/HDL FIFO3/Upsample2/Counter</item>
  | 				</Source>
  | 			</first>
  | 			<second>
  | 				<SuppressedData>
  | 					<count>2</count>
  | 					<bucket_count>2</bucket_count>
  | 					<item_version>0</item_version>
  | 					<item>
  | 						<first>
  | 							<ID>Simulink:DataType:WarningOverFlowDetected</ID>
  | 							<Cause>
  | 								<Source>
  | 									<count>0</count>
  | 									<item_version>0</item_version>
  | 								</Source>
  | 							</Cause>
  | 						</first>
  | 						<second>
  | 							<Comment></Comment>
  | 							<User></User>
  | 							<LastModified>
  | 								<ptime_date>
  | 									<date>20160608</date>
  | 								</ptime_date>
  | 								<ptime_time_duration>
  | 									<is_special>0</is_special>
  | 									<time_duration_hours>15</time_duration_hours>
  | 									<time_duration_minutes>23</time_duration_minutes>
  | 									<time_duration_seconds>17</time_duration_seconds>
  | 									<time_duration_fractional_seconds>0</time_duration_fractional_seconds>
  | 								</ptime_time_duration>
  | 							</LastModified>
  | 							<SuppressionType>1</SuppressionType>
  | 						</second>
  | 					</item>
  | 					<item>
  | 						<first>
  | 							<ID>SimulinkFixedPoint:util:Overflowoccurred</ID>
  | 							<Cause>
  | 								<Source>
  | 									<count>0</count>
  | 									<item_version>0</item_version>
  | 								</Source>
  | 							</Cause>
  | 						</first>
  | 						<second>
  | 							<Comment></Comment>
  | 							<User></User>
  | 							<LastModified>
  | 								<ptime_date>
  | 									<date>20160608</date>
  | 								</ptime_date>
  | 								<ptime_time_duration>
  | 									<is_special>0</is_special>
  | 									<time_duration_hours>15</time_duration_hours>
  | 									<time_duration_minutes>23</time_duration_minutes>
  | 									<time_duration_seconds>17</time_duration_seconds>
  | 									<time_duration_fractional_seconds>0</time_duration_fractional_seconds>
  | 								</ptime_time_duration>
  | 							</LastModified>
  | 							<SuppressionType>1</SuppressionType>
  | 						</second>
  | 					</item>
  | 				</SuppressedData>
  | 			</second>
  | 		</item>
  | 		<item>
  | 			<first>
  | 				<Source>
  | 					<count>1</count>
  | 					<item_version>0</item_version>
  | 					<item>RxTxFixedPointLibrary_noscopes_org/Receiver HDL/Frame Recover/Equalization and Demodulation/DFE/Packeted To Unpacked/Extract Bits</item>
  | 				</Source>
  | 			</first>
  | 			<second>
  | 				<SuppressedData>
  | 					<count>2</count>
  | 					<bucket_count>2</bucket_count>
  | 					<item_version>0</item_version>
  | 					<item>
  | 						<first>
  | 							<ID>SimulinkFixedPoint:util:Overflowoccurred</ID>
  | 							<Cause>
  | 								<Source>
  | 									<count>0</count>
  | 									<item_version>0</item_version>
  | 								</Source>
  | 							</Cause>
  | 						</first>
  | 						<second>
  | 							<Comment></Comment>
  | 							<User></User>
  | 							<LastModified>
  | 								<ptime_date>
  | 									<date>20160608</date>
  | 								</ptime_date>
  | 								<ptime_time_duration>
  | 									<is_special>0</is_special>
  | 									<time_duration_hours>15</time_duration_hours>
  | 									<time_duration_minutes>43</time_duration_minutes>
  | 									<time_duration_seconds>6</time_duration_seconds>
  | 									<time_duration_fractional_seconds>0</time_duration_fractional_seconds>
  | 								</ptime_time_duration>
  | 							</LastModified>
  | 							<SuppressionType>1</SuppressionType>
  | 						</second>
  | 					</item>
  | 					<item>
  | 						<first>
  | 							<ID>Simulink:DataType:WarningOverFlowDetected</ID>
  | 							<Cause>
  | 								<Source>
  | 									<count>0</count>
  | 									<item_version>0</item_version>
  | 								</Source>
  | 							</Cause>
  | 						</first>
  | 						<second>
  | 							<Comment></Comment>
  | 							<User></User>
  | 							<LastModified>
  | 								<ptime_date>
  | 									<date>20160608</date>
  | 								</ptime_date>
  | 								<ptime_time_duration>
  | 									<is_special>0</is_special>
  | 									<time_duration_hours>15</time_duration_hours>
  | 									<time_duration_minutes>43</time_duration_minutes>
  | 									<time_duration_seconds>6</time_duration_seconds>
  | 									<time_duration_fractional_seconds>0</time_duration_fractional_seconds>
  | 								</ptime_time_duration>
  | 							</LastModified>
  | 							<SuppressionType>1</SuppressionType>
  | 						</second>
  | 					</item>
  | 				</SuppressedData>
  | 			</second>
  | 		</item>
  | 		<item>
  | 			<first>
  | 				<Source>
  | 					<count>1</count>
  | 					<item_version>0</item_version>
  | 					<item>RxTxFixedPointLibrary_noscopes_org/Receiver HDL/Frame Recover/Frequency Recovery/Phase Shift FP/Cosine HDL Optimized/exp hdl/sin_hdl</item>
  | 				</Source>
  | 			</first>
  | 			<second>
  | 				<SuppressedData>
  | 					<count>1</count>
  | 					<bucket_count>2</bucket_count>
  | 					<item_version>0</item_version>
  | 					<item>
  | 						<first>
  | 							<ID>SimulinkFixedPoint:util:fxpParameterPrecisionLoss</ID>
  | 							<Cause>
  | 								<Source>
  | 									<count>0</count>
  | 									<item_version>0</item_version>
  | 								</Source>
  | 							</Cause>
  | 						</first>
  | 						<second>
  | 							<Comment></Comment>
  | 							<User></User>
  | 							<LastModified>
  | 								<ptime_date>
  | 									<date>20160607</date>
  | 								</ptime_date>
  | 								<ptime_time_duration>
  | 									<is_special>0</is_special>
  | 									<time_duration_hours>13</time_duration_hours>
  | 									<time_duration_minutes>40</time_duration_minutes>
  | 									<time_duration_seconds>50</time_duration_seconds>
  | 									<time_duration_fractional_seconds>0</time_duration_fractional_seconds>
  | 								</ptime_time_duration>
  | 							</LastModified>
  | 							<SuppressionType>1</SuppressionType>
  | 						</second>
  | 					</item>
  | 				</SuppressedData>
  | 			</second>
  | 		</item>
  | 		<item>
  | 			<first>
  | 				<Source>
  | 					<count>1</count>
  | 					<item_version>0</item_version>
  | 					<item>RxTxFixedPointLibrary_noscopes_org/Receiver HDL/Frame Recover/Equalization and Demodulation/DFE/Packeted To Unpacked/Extract Bits1</item>
  | 				</Source>
  | 			</first>
  | 			<second>
  | 				<SuppressedData>
  | 					<count>2</count>
  | 					<bucket_count>2</bucket_count>
  | 					<item_version>0</item_version>
  | 					<item>
  | 						<first>
  | 							<ID>SimulinkFixedPoint:util:Overflowoccurred</ID>
  | 							<Cause>
  | 								<Source>
  | 									<count>0</count>
  | 									<item_version>0</item_version>
  | 								</Source>
  | 							</Cause>
  | 						</first>
  | 						<second>
  | 							<Comment></Comment>
  | 							<User></User>
  | 							<LastModified>
  | 								<ptime_date>
  | 									<date>20160608</date>
  | 								</ptime_date>
  | 								<ptime_time_duration>
  | 									<is_special>0</is_special>
  | 									<time_duration_hours>15</time_duration_hours>
  | 									<time_duration_minutes>43</time_duration_minutes>
  | 									<time_duration_seconds>6</time_duration_seconds>
  | 									<time_duration_fractional_seconds>0</time_duration_fractional_seconds>
  | 								</ptime_time_duration>
  | 							</LastModified>
  | 							<SuppressionType>1</SuppressionType>
  | 						</second>
  | 					</item>
  | 					<item>
  | 						<first>
  | 							<ID>Simulink:DataType:WarningOverFlowDetected</ID>
  | 							<Cause>
  | 								<Source>
  | 									<count>0</count>
  | 									<item_version>0</item_version>
  | 								</Source>
  | 							</Cause>
  | 						</first>
  | 						<second>
  | 							<Comment></Comment>
  | 							<User></User>
  | 							<LastModified>
  | 								<ptime_date>
  | 									<date>20160608</date>
  | 								</ptime_date>
  | 								<ptime_time_duration>
  | 									<is_special>0</is_special>
  | 									<time_duration_hours>15</time_duration_hours>
  | 									<time_duration_minutes>43</time_duration_minutes>
  | 									<time_duration_seconds>6</time_duration_seconds>
  | 									<time_duration_fractional_seconds>0</time_duration_fractional_seconds>
  | 								</ptime_time_duration>
  | 							</LastModified>
  | 							<SuppressionType>1</SuppressionType>
  | 						</second>
  | 					</item>
  | 				</SuppressedData>
  | 			</second>
  | 		</item>
  | 	</Table>
  | </DiagnosticSuppressor>
  | </boost_serialization>

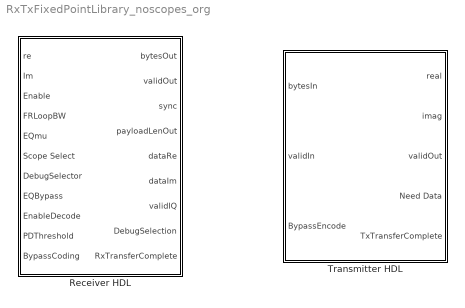
== system RxTxFixedPointLibrary_noscopes_org ==
  Receiver HDL : Subsystem  TreatAsAtomicUnit=on
      mask Display:
      | if ispc
      |     d = '\';
      | else
      |     d = '/';
      | end
      | model_path = get_param(bdroot, 'FileName');
      | %info = Simulink.MDLInfo(bdroot)
      | c = strsplit(model_path,d); c = strjoin(c(1:end-2),d);
      | logo = [c,d,'ADI_logo.svg'];
      | %disp(logo);
      | image(logo);
  Transmitter HDL : Subsystem  TreatAsAtomicUnit=on
      mask Display:
      | if ispc
      |     d = '\';
      | else
      |     d = '/';
      | end
      | model_path = get_param(bdroot, 'FileName');
      | %info = Simulink.MDLInfo(bdroot)
      | c = strsplit(model_path,d); c = strjoin(c(1:end-2),d);
      | logo = [c,d,'ADI_logo.svg'];
      | %disp(logo);
      | image(logo);
